simulink library "CryoDetLibCMB"  (R2016b)
settings: Solver=VariableStepAuto  StartTime=0.0  StopTime=10.0  RelTol=1e-3
undefined symbols (not defined in the file): A, B, C, D, Fadc, Fclk, PCIN, xlipgetpartsetting
libraries: xbsIndex_r4 x640, CryoDetLibCMB x81, CryoDetLib x2, simulink x1
(part 6 of 12)

== system CryoDetLibCMB/DDS 8ch ==
  note: don't worry about matching latency here, will do downstream
  note: 8 Channel DDS
      | Given its channel ID, takes instantaneous frequency for this channel of each band and generates phase and I&Q
      | interleaved over 8 bands
      | Frequency RAM is updated asynchronously to operation
  note: Phase Accumulator
      | (8 Channels)
  note: Frequency RAM
  note: Sinc/Cos Generator
  valid : Inport
  freqWord : Inport  Port=2
  index : Inport  Port=3
  ch : Inport  Port=4
  AddSub : xbsIndex_r4/AddSub  mode=Addition  use_carryin=off  use_carryout=off  en=off  latency=3  precision=User Defined  arith_type=Unsigned  n_bits=24  bin_pt=24  quantization=Truncate  overflow=Wrap  use_behavioral_HDL=off  hw_selection=Fabric  pipelined=off  dbl_ovrd=off  block_type=addsub
  BitBasher : xbsIndex_r4/BitBasher  bitexpr=|  display_expr=off  sr_1=tmux  arith_type1=Unsigned  bin_pt1=0  sr_2=subband  arith_type2=Unsigned  bin_pt2=0  sr_3=3  arith_type3=Unsigned  bin_pt3=0  sr_4=4  arith_type4=Unsigned  bin_pt4=0  dbl_ovrd=off  block_type=bitbasher
      | tmux = {in[6:4]}
      | subband = {in[3:0]}
  BitBasher1 : xbsIndex_r4/BitBasher  bitexpr=|  display_expr=off  sr_1=ch  arith_type1=Unsigned  bin_pt1=0  sr_2=amp  arith_type2=Unsigned  bin_pt2=0  sr_3=3  arith_type3=Unsigned  bin_pt3=0  sr_4=4  arith_type4=Unsigned  bin_pt4=0  dbl_ovrd=off  block_type=bitbasher
      | ch = {in[6:4]}
      | amp = {in[3:0]}
  BitBasher2 : xbsIndex_r4/BitBasher  bitexpr=|  display_expr=off  sr_1=freq  arith_type1=Unsigned  bin_pt1=24  sr_2=amp  arith_type2=Unsigned  bin_pt2=0  sr_3=3  arith_type3=Unsigned  bin_pt3=0  sr_4=4  arith_type4=Unsigned  bin_pt4=0  dbl_ovrd=off  block_type=bitbasher
      | freq = {in[23:0]}
      | amp = {in[27:24]}
  BitBasher3 : xbsIndex_r4/BitBasher  bitexpr=out = {ch, amp}  display_expr=off  sr_1=out  arith_type1=Unsigned  bin_pt1=0  sr_2=amp  arith_type2=Unsigned  bin_pt2=0  sr_3=3  arith_type3=Unsigned  bin_pt3=0  sr_4=4  arith_type4=Unsigned  bin_pt4=0  dbl_ovrd=off  block_type=bitbasher
  BitBasher4 : xbsIndex_r4/BitBasher  bitexpr=|  display_expr=off  sr_1=ch  arith_type1=Unsigned  bin_pt1=0  sr_2=amp  arith_type2=Unsigned  bin_pt2=0  sr_3=3  arith_type3=Unsigned  bin_pt3=0  sr_4=4  arith_type4=Unsigned  bin_pt4=0  dbl_ovrd=off  block_type=bitbasher
      | ch = {in[6:4]}
      | amp = {in[3:0]}
  Bus Creator : BusCreator  Inputs=3
  Convert : xbsIndex_r4/Convert  gui_display_data_type=Fixed-point  arith_type=Unsigned  n_bits=14  bin_pt=14  float_type=Single  exp_bits=8  fraction_bits=24  quantization=Truncate  overflow=Wrap  en=off  latency=1  pipeline=off  dbl_ovrd=off  block_type=convert
  Counter : xbsIndex_r4/Counter  cnt_type=Free Running  cnt_to=Inf  operation=Up  start_count=0  cnt_by_val=1  arith_type=Unsigned  n_bits=3  bin_pt=0  load_pin=off  rst=off  en=on  explicit_period=off  period=1  use_behavioral_HDL=off  implementation=Fabric  dbl_ovrd=off  block_type=counter
  "DDS Compiler 6.0 " : xbsIndex_r4/DDS Compiler 6.0   partspresent=SIN_COS_LUT_only  dds_clock_rate=100  channels=1  mode_of_operation=Standard  modulus=9  parameter_entry=System_Parameters  spurious_free_dynamic_range=45  frequency_resolution=0.4  noise_shaping=None  phase_width=14  output_width=16  output_selection=Sine_and_Cosine  negative_sine=off  negative_cosine=off  amplitude_mode=Full_Range  memory_type=Auto  optimization_goal=Auto  dsp48_use=Minimal  resync=off  latency_configuration=Auto  latency=1  has_phase_out=off  has_aclken=off  has_aresetn=off  explicit_period=off  period=1  data_has_tlast=Not_Required  has_tready=off  s_phase_has_tuser=User_Field  m_data_has_tuser=User_Field  m_phase_has_tuser=Not_Required  s_phase_tuser_width=7  output_form=Twos_Complement  s_config_sync_mode=On_Vector  phase_increment=Streaming  output_frequency1=0  output_frequency2=0  output_frequency3=0  output_frequency4=0  output_frequency5=0  output_frequency6=0  output_frequency7=0  output_frequency8=0  output_frequency9=0  output_frequency10=0  output_frequency11=0  output_frequency12=0  output_frequency13=0  output_frequency14=0  output_frequency15=0  output_frequency16=0  pinc1='0'  pinc2='0'  pinc3='0'  pinc4='0'  pinc5='0'  pinc6='0'  pinc7='0'  pinc8='0'  pinc9='0'  pinc10='0'  pinc11='0'  pinc12='0'  pinc13='0'  pinc14='0'  pinc15='0'  pinc16='0'  phase_offset=Streaming  phase_offset_angles1=0  phase_offset_angles2=0  phase_offset_angles3=0  phase_offset_angles4=0  phase_offset_angles5=0  phase_offset_angles6=0  phase_offset_angles7=0  phase_offset_angles8=0  phase_offset_angles9=0  phase_offset_angles10=0  phase_offset_angles11=0  phase_offset_angles12=0  phase_offset_angles13=0  phase_offset_angles14=0  phase_offset_angles15=0  phase_offset_angles16=0  poff1='0'  poff2='0'  poff3='0'  poff4='0'  poff5='0'  poff6='0'  poff7='0'  poff8='0'  poff9='0'  poff10='0'  poff11='0'  poff12='0'  poff13='0'  poff14='0'  poff15='0'  poff16='0'  trim_axipin_name=on  simulation_type=hybrid_sim  simulation_model=sysgen:xddsv6_0_cmodel  data_path_portlist={ 's_axis_config_tdata_poff', 's_axis_config_tdata_chan0_poff', 's_axis_config_tdata_pinc', 's_axis_config_tdata_chan0_pinc', 's_axis_phase_tdata_resync', 's_axis_phase_tdata_chan0_resync', 's_axis_phase_tdata_poff', 's_axis_phase_tdata_chan0_poff', 's_axis_phase_tdata_pinc', 's_axis_phase_tdata_chan0_pinc', 's_axis_phase_tdata_phase_in', 'm_axis_data_tdata_sine', 'm_axis_data_tdata_chan0_sine', 'm_axis_data_tdata_cosine', 'm_axis_data_tdata_chan0_cosine', 'm_axis_phase_tdata_phase_out', 'm_axis_phase_tdata_chan0_phase_out'}  por_mode=false  gui_behaviour=Sysgen  ip_name=DDS Compiler  ip_version=6.0  dsptool_ready=true  wrapper_available=true  port_translation_map={ 'aclken' => 'en', 'aresetn' => 'rst' }  ipcore_usecache=true  ipcore_useipmodelcache=true  ipcore_xco_need_fpga_part=true  ipcore_verbose=false  block_type=dds_compiler_v6_0
  Delay : xbsIndex_r4/Delay  rst=off  infoeditControl=Selection of Reset will increase slice count due to use of real FFs and instead of SRLs  en=off  latency=5  reg_retiming=off  dbl_ovrd=off  block_type=delay
  Delay1 : xbsIndex_r4/Delay  rst=off  infoeditControl=Selection of Reset will increase slice count due to use of real FFs and instead of SRLs  en=off  latency=4  reg_retiming=off  dbl_ovrd=off  block_type=delay
  Delay2 : xbsIndex_r4/Delay  rst=off  infoeditControl=Selection of Reset will increase slice count due to use of real FFs and instead of SRLs  en=off  latency=2  reg_retiming=off  dbl_ovrd=off  block_type=delay
  Delay4 : xbsIndex_r4/Delay  rst=off  infoeditControl=Selection of Reset will increase slice count due to use of real FFs and instead of SRLs  en=off  latency=6  reg_retiming=off  dbl_ovrd=off  block_type=delay
  Dual Port RAM : xbsIndex_r4/Dual Port RAM  depth=8  initVector=0  distributed_mem=Distributed memory  init_a=0  init_b=0  rst_a=off  rst_b=off  en_a=off  en_b=off  latency=1  write_mode_A=Read After Write  write_mode_B=Read After Write  optimize=Area  dbl_ovrd=off  block_type=dpram
  Register{,1..2,6} (4 alike) : xbsIndex_r4/Register  init=0  rst=off  en=off  dbl_ovrd=off  block_type=register
  Register3 : xbsIndex_r4/Register  init=0  rst=off  en=on  dbl_ovrd=off  block_type=register
  Register4 : xbsIndex_r4/Register  init=0  rst=off  en=on  dbl_ovrd=off  block_type=register
  Register5 : xbsIndex_r4/Register  init=0  rst=off  en=on  dbl_ovrd=off  block_type=register
  Relational : xbsIndex_r4/Relational  mode=a=b  op_type=Bool  en=off  latency=1  dbl_ovrd=off  block_type=relational
  Terminator : Terminator
  valid1 : InportShadow
  valid_o : Outport
  Q : Outport  Port=2
  I : Outport  Port=3
  amp_o : Outport  Port=4
  ch_o : Outport  Port=5
  phaseBus : Outport  Port=6
  wires:
  BitBasher1/1 -> Bus Creator/3  "ch"
  BitBasher4/2 -> amp_o/1
  "DDS Compiler 6.0 "/4 -> Register5/1  "INDX"
  "DDS Compiler 6.0 "/3 -> Register4/1  "I"
  Counter/1 -> Dual Port RAM/4, Delay2/1
  valid1/1 -> Delay4/1
  valid/1 -> Counter/1
  Delay4/1 -> Bus Creator/1, "DDS Compiler 6.0 "/1  "valid"
  "DDS Compiler 6.0 "/1 -> Register2/1, Register5/2, Register4/2, Register3/2  "valid"
  "DDS Compiler 6.0 "/2 -> Register3/1  "Q"
  Register1/1 -> Dual Port RAM/2
  Register/1 -> Dual Port RAM/1
  Delay1/1 -> BitBasher1/1, "DDS Compiler 6.0 "/3  "ch"
  Dual Port RAM/1 -> Terminator/1
  Convert/1 -> Bus Creator/2, "DDS Compiler 6.0 "/2  "phase"
  AddSub/1 -> Convert/1, Delay/1
  ch/1 -> BitBasher/1
  Delay/1 -> AddSub/1
  Relational/1 -> Dual Port RAM/3
  BitBasher/1 -> Register/1
  BitBasher/2 -> Relational/1
  index/1 -> Relational/2
  Register4/1 -> I/1  "I"
  Register3/1 -> Q/1  "Q"
  Register2/1 -> valid_o/1  "valid"
  freqWord/1 -> Register1/1
  Dual Port RAM/2 -> Register6/1
  BitBasher2/1 -> AddSub/2
  BitBasher2/2 -> BitBasher3/1
  BitBasher3/1 -> Delay1/1
  Register5/1 -> BitBasher4/1  "INDX"
  BitBasher4/1 -> ch_o/1
  Register6/1 -> BitBasher2/1
  Delay2/1 -> BitBasher3/2
  Bus Creator/1 -> phaseBus/1

== system CryoDetLibCMB/DDS 8ch taylor series corrected ==
  note: Taylor series corrected - use 0.5 BRAM (18 bit storage, 2^10 points), 3DSP
  note: Frequency RAM
  note: Phase Accumulator
      | (8 Channels)
  note: 8 Channel DDS
      | Given its channel ID, takes instantaneous frequency for this channel of each band and generates phase and I&Q
      | interleaved over 8 bands
      | Frequency RAM is updated asynchronously to operation
  note: don't worry about matching latency here, will do downstream
  valid : Inport
  rst : Inport  Port=2
  freqWord : Inport  Port=3
  index : Inport  Port=4
  ch : Inport  Port=5
  BitBasher : xbsIndex_r4/BitBasher  bitexpr=|  display_expr=off  sr_1=tmux  arith_type1=Unsigned  bin_pt1=0  sr_2=subband  arith_type2=Unsigned  bin_pt2=0  sr_3=3  arith_type3=Unsigned  bin_pt3=0  sr_4=4  arith_type4=Unsigned  bin_pt4=0  dbl_ovrd=off  block_type=bitbasher
      | tmux = {in[6:4]}
      | subband = {in[3:0]}
  BitBasher1 : xbsIndex_r4/BitBasher  bitexpr=|  display_expr=off  sr_1=ch  arith_type1=Unsigned  bin_pt1=0  sr_2=amp  arith_type2=Unsigned  bin_pt2=0  sr_3=3  arith_type3=Unsigned  bin_pt3=0  sr_4=4  arith_type4=Unsigned  bin_pt4=0  dbl_ovrd=off  block_type=bitbasher
      | ch = {in[6:4]}
      | amp = {in[3:0]}
  BitBasher2 : xbsIndex_r4/BitBasher  bitexpr=|  display_expr=off  sr_1=freq  arith_type1=Unsigned  bin_pt1=24  sr_2=amp  arith_type2=Unsigned  bin_pt2=0  sr_3=3  arith_type3=Unsigned  bin_pt3=0  sr_4=4  arith_type4=Unsigned  bin_pt4=0  dbl_ovrd=off  block_type=bitbasher
      | freq = {in[23:0]}
      | amp = {in[27:24]}
  BitBasher3 : xbsIndex_r4/BitBasher  bitexpr=out = {ch, amp}  display_expr=off  sr_1=out  arith_type1=Unsigned  bin_pt1=0  sr_2=amp  arith_type2=Unsigned  bin_pt2=0  sr_3=3  arith_type3=Unsigned  bin_pt3=0  sr_4=4  arith_type4=Unsigned  bin_pt4=0  dbl_ovrd=off  block_type=bitbasher
  BitBasher4 : xbsIndex_r4/BitBasher  bitexpr=|  display_expr=off  sr_1=ch  arith_type1=Unsigned  bin_pt1=0  sr_2=amp  arith_type2=Unsigned  bin_pt2=0  sr_3=3  arith_type3=Unsigned  bin_pt3=0  sr_4=4  arith_type4=Unsigned  bin_pt4=0  dbl_ovrd=off  block_type=bitbasher
      | ch = {in[6:4]}
      | amp = {in[3:0]}
  BitBasher5 : xbsIndex_r4/BitBasher  bitexpr=phase = {in[23:8]}  display_expr=off  sr_1=phase  arith_type1="Signed  (2's comp)"  bin_pt1=15  sr_2=amp  arith_type2=Unsigned  bin_pt2=0  sr_3=3  arith_type3=Unsigned  bin_pt3=0  sr_4=4  arith_type4=Unsigned  bin_pt4=0  dbl_ovrd=off  block_type=bitbasher
  Bus Creator : BusCreator  Inputs=3
  Counter : xbsIndex_r4/Counter  cnt_type=Free Running  cnt_to=Inf  operation=Up  start_count=0  cnt_by_val=1  arith_type=Unsigned  n_bits=3  bin_pt=0  load_pin=off  rst=on  en=on  explicit_period=off  period=1  use_behavioral_HDL=off  implementation=Fabric  dbl_ovrd=off  block_type=counter
  DDS Compiler 6.0 1 : xbsIndex_r4/DDS Compiler 6.0   partspresent=Phase_Generator_only  dds_clock_rate=100  channels=8  mode_of_operation=Standard  modulus=9  parameter_entry=System_Parameters  spurious_free_dynamic_range=45  frequency_resolution=0.4  noise_shaping=None  phase_width=24  output_width=3  output_selection=Sine_and_Cosine  negative_sine=off  negative_cosine=off  amplitude_mode=Full_Range  memory_type=Auto  optimization_goal=Auto  dsp48_use=Minimal  resync=off  latency_configuration=Auto  latency=1  has_phase_out=on  has_aclken=off  has_aresetn=on  explicit_period=off  period=1  data_has_tlast=Not_Required  has_tready=off  s_phase_has_tuser=User_Field  m_data_has_tuser=Not_Required  m_phase_has_tuser=User_Field  s_phase_tuser_width=7  output_form=Twos_Complement  s_config_sync_mode=On_Vector  phase_increment=Streaming  output_frequency1=0  output_frequency2=0  output_frequency3=0  output_frequency4=0  output_frequency5=0  output_frequency6=0  output_frequency7=0  output_frequency8=0  output_frequency9=0  output_frequency10=0  output_frequency11=0  output_frequency12=0  output_frequency13=0  output_frequency14=0  output_frequency15=0  output_frequency16=0  pinc1='0'  pinc2='0'  pinc3='0'  pinc4='0'  pinc5='0'  pinc6='0'  pinc7='0'  pinc8='0'  pinc9='0'  pinc10='0'  pinc11='0'  pinc12='0'  pinc13='0'  pinc14='0'  pinc15='0'  pinc16='0'  phase_offset=None  phase_offset_angles1=0  phase_offset_angles2=0  phase_offset_angles3=0  phase_offset_angles4=0  phase_offset_angles5=0  phase_offset_angles6=0  phase_offset_angles7=0  phase_offset_angles8=0  phase_offset_angles9=0  phase_offset_angles10=0  phase_offset_angles11=0  phase_offset_angles12=0  phase_offset_angles13=0  phase_offset_angles14=0  phase_offset_angles15=0  phase_offset_angles16=0  poff1='0'  poff2='0'  poff3='0'  poff4='0'  poff5='0'  poff6='0'  poff7='0'  poff8='0'  poff9='0'  poff10='0'  poff11='0'  poff12='0'  poff13='0'  poff14='0'  poff15='0'  poff16='0'  trim_axipin_name=on  simulation_type=hybrid_sim  simulation_model=sysgen:xddsv6_0_cmodel  data_path_portlist={ 's_axis_config_tdata_poff', 's_axis_config_tdata_chan0_poff', 's_axis_config_tdata_pinc', 's_axis_config_tdata_chan0_pinc', 's_axis_phase_tdata_resync', 's_axis_phase_tdata_chan0_resync', 's_axis_phase_tdata_poff', 's_axis_phase_tdata_chan0_poff', 's_axis_phase_tdata_pinc', 's_axis_phase_tdata_chan0_pinc', 's_axis_phase_tdata_phase_in', 'm_axis_data_tdata_sine', 'm_axis_data_tdata_chan0_sine', 'm_axis_data_tdata_cosine', 'm_axis_data_tdata_chan0_cosine', 'm_axis_phase_tdata_phase_out', 'm_axis_phase_tdata_chan0_phase_out'}  por_mode=false  gui_behaviour=Sysgen  ip_name=DDS Compiler  ip_version=6.0  dsptool_ready=true  wrapper_available=true  port_translation_map={ 'aclken' => 'en', 'aresetn' => 'rst' }  ipcore_usecache=true  ipcore_useipmodelcache=true  ipcore_xco_need_fpga_part=true  ipcore_verbose=false  block_type=dds_compiler_v6_0
  DDS Compiler 6.0 2 : xbsIndex_r4/DDS Compiler 6.0   partspresent=SIN_COS_LUT_only  dds_clock_rate=100  channels=1  mode_of_operation=Standard  modulus=9  parameter_entry=System_Parameters  spurious_free_dynamic_range=45  frequency_resolution=0.4  noise_shaping=Taylor_Series_Corrected  phase_width=24  output_width=18  output_selection=Sine_and_Cosine  negative_sine=off  negative_cosine=off  amplitude_mode=Full_Range  memory_type=Auto  optimization_goal=Area  dsp48_use=Minimal  resync=off  latency_configuration=Auto  latency=1  has_phase_out=off  has_aclken=off  has_aresetn=off  explicit_period=off  period=1  data_has_tlast=Not_Required  has_tready=off  s_phase_has_tuser=User_Field  m_data_has_tuser=User_Field  m_phase_has_tuser=Not_Required  s_phase_tuser_width=7  output_form=Twos_Complement  s_config_sync_mode=On_Vector  phase_increment=Streaming  output_frequency1=0  output_frequency2=0  output_frequency3=0  output_frequency4=0  output_frequency5=0  output_frequency6=0  output_frequency7=0  output_frequency8=0  output_frequency9=0  output_frequency10=0  output_frequency11=0  output_frequency12=0  output_frequency13=0  output_frequency14=0  output_frequency15=0  output_frequency16=0  pinc1='0'  pinc2='0'  pinc3='0'  pinc4='0'  pinc5='0'  pinc6='0'  pinc7='0'  pinc8='0'  pinc9='0'  pinc10='0'  pinc11='0'  pinc12='0'  pinc13='0'  pinc14='0'  pinc15='0'  pinc16='0'  phase_offset=Streaming  phase_offset_angles1=0  phase_offset_angles2=0  phase_offset_angles3=0  phase_offset_angles4=0  phase_offset_angles5=0  phase_offset_angles6=0  phase_offset_angles7=0  phase_offset_angles8=0  phase_offset_angles9=0  phase_offset_angles10=0  phase_offset_angles11=0  phase_offset_angles12=0  phase_offset_angles13=0  phase_offset_angles14=0  phase_offset_angles15=0  phase_offset_angles16=0  poff1='0'  poff2='0'  poff3='0'  poff4='0'  poff5='0'  poff6='0'  poff7='0'  poff8='0'  poff9='0'  poff10='0'  poff11='0'  poff12='0'  poff13='0'  poff14='0'  poff15='0'  poff16='0'  trim_axipin_name=on  simulation_type=hybrid_sim  simulation_model=sysgen:xddsv6_0_cmodel  data_path_portlist={ 's_axis_config_tdata_poff', 's_axis_config_tdata_chan0_poff', 's_axis_config_tdata_pinc', 's_axis_config_tdata_chan0_pinc', 's_axis_phase_tdata_resync', 's_axis_phase_tdata_chan0_resync', 's_axis_phase_tdata_poff', 's_axis_phase_tdata_chan0_poff', 's_axis_phase_tdata_pinc', 's_axis_phase_tdata_chan0_pinc', 's_axis_phase_tdata_phase_in', 'm_axis_data_tdata_sine', 'm_axis_data_tdata_chan0_sine', 'm_axis_data_tdata_cosine', 'm_axis_data_tdata_chan0_cosine', 'm_axis_phase_tdata_phase_out', 'm_axis_phase_tdata_chan0_phase_out'}  por_mode=false  gui_behaviour=Sysgen  ip_name=DDS Compiler  ip_version=6.0  dsptool_ready=true  wrapper_available=true  port_translation_map={ 'aclken' => 'en', 'aresetn' => 'rst' }  ipcore_usecache=true  ipcore_useipmodelcache=true  ipcore_xco_need_fpga_part=true  ipcore_verbose=false  block_type=dds_compiler_v6_0
  Delay2 : xbsIndex_r4/Delay  rst=off  infoeditControl=Selection of Reset will increase slice count due to use of real FFs and instead of SRLs  en=off  latency=2  reg_retiming=off  dbl_ovrd=off  block_type=delay
  Delay4 : xbsIndex_r4/Delay  rst=off  infoeditControl=Selection of Reset will increase slice count due to use of real FFs and instead of SRLs  en=off  latency=2  reg_retiming=off  dbl_ovrd=off  block_type=delay
  Dual Port RAM : xbsIndex_r4/Dual Port RAM  depth=8  initVector=0  distributed_mem=Distributed memory  init_a=0  init_b=0  rst_a=off  rst_b=off  en_a=off  en_b=off  latency=1  write_mode_A=Read After Write  write_mode_B=Read After Write  optimize=Area  dbl_ovrd=off  block_type=dpram
  Inverter : xbsIndex_r4/Inverter  en=off  latency=1  dbl_ovrd=off  block_type=inv
  Register{,1..2,6} (4 alike) : xbsIndex_r4/Register  init=0  rst=off  en=off  dbl_ovrd=off  block_type=register
  Register3 : xbsIndex_r4/Register  init=0  rst=off  en=on  dbl_ovrd=off  block_type=register
  Register4 : xbsIndex_r4/Register  init=0  rst=off  en=on  dbl_ovrd=off  block_type=register
  Register5 : xbsIndex_r4/Register  init=0  rst=off  en=on  dbl_ovrd=off  block_type=register
  Relational : xbsIndex_r4/Relational  mode=a=b  op_type=Bool  en=off  latency=1  dbl_ovrd=off  block_type=relational
  Terminator : Terminator
  Terminator1 : Terminator
  Terminator2 : Terminator
  tuser : xbsIndex_r4/Constant  const=0  gui_display_data_type=Boolean  arith_type=Boolean  n_bits=1  bin_pt=0  preci_type=Single  exp_width=8  frac_width=24  explicit_period=off  period=1  equ=P=C  opselect=C  inp2=PCIN>>17  opr=+  inp1=P  carry=CIN  dbl_ovrd=off  block_type=constant
  valid1 : InportShadow
  valid_o : Outport
  Q : Outport  Port=2
  I : Outport  Port=3
  amp_o : Outport  Port=4
  ch_o : Outport  Port=5
  phaseBus : Outport  Port=6
  wires:
  Inverter/1 -> DDS Compiler 6.0 1/5
  valid/1 -> Counter/2
  rst/1 -> Counter/1, Inverter/1
  BitBasher5/1 -> Bus Creator/2  "phase"
  Bus Creator/1 -> phaseBus/1
  Delay2/1 -> BitBasher3/2
  Register6/1 -> BitBasher2/1
  BitBasher4/1 -> ch_o/1
  Register5/1 -> BitBasher4/1  "INDX"
  BitBasher2/2 -> BitBasher3/1
  Dual Port RAM/2 -> Register6/1
  freqWord/1 -> Register1/1
  Register2/1 -> valid_o/1  "valid"
  Register3/1 -> Q/1  "Q"
  Register4/1 -> I/1  "I"
  index/1 -> Relational/2
  BitBasher/2 -> Relational/1
  BitBasher/1 -> Register/1
  Relational/1 -> Dual Port RAM/3
  ch/1 -> BitBasher/1
  Dual Port RAM/1 -> Terminator/1
  Register/1 -> Dual Port RAM/1
  Register1/1 -> Dual Port RAM/2
  DDS Compiler 6.0 2/2 -> Register3/1  "Q"
  DDS Compiler 6.0 2/1 -> Register5/2, Register4/2, Register3/2, Register2/1  "valid"
  valid1/1 -> Delay4/1
  Counter/1 -> Delay2/1, Dual Port RAM/4
  DDS Compiler 6.0 2/3 -> Register4/1  "I"
  DDS Compiler 6.0 2/4 -> Register5/1  "INDX"
  BitBasher4/2 -> amp_o/1
  BitBasher1/1 -> Bus Creator/3  "ch"
  DDS Compiler 6.0 1/1 -> Bus Creator/1, DDS Compiler 6.0 2/1  "valid"
  BitBasher2/1 -> DDS Compiler 6.0 1/2
  BitBasher3/1 -> DDS Compiler 6.0 1/4
  Delay4/1 -> DDS Compiler 6.0 1/1  "valid"
  DDS Compiler 6.0 1/2 -> DDS Compiler 6.0 2/2, BitBasher5/1  "phase"
  DDS Compiler 6.0 1/3 -> DDS Compiler 6.0 2/3, BitBasher1/1  "tyser"
  tuser/1 -> DDS Compiler 6.0 1/3
  DDS Compiler 6.0 1/4 -> Terminator1/1
  DDS Compiler 6.0 1/5 -> Terminator2/1

== system CryoDetLibCMB/DDS Mixer ==
  In : Inport
  freqBus : Inport  Port=2
  index : Inport  Port=3
  Bus Creator1 : BusCreator  Inputs=4
  Bus Creator2 : BusCreator  Inputs=5
  Bus Selector1 : BusSelector  OutputSignals=valid,Q,I,amp,ch
  Bus Selector2 : BusSelector  OutputSignals=valid
  Bus Selector : BusSelector  OutputSignals=freqWord,ch
  DDS 8ch : CryoDetLibCMB/DDS 8ch
  IQ_scale : CryoDetLibCMB/IQ_scale
  mixer : Subsystem
  tones : Outport
  downconvert : Outport  Port=2
  phase : Outport  Port=3
  wires:
  Bus Selector/1 -> DDS 8ch/2  "<freqWord>"
  Bus Selector1/5 -> IQ_scale/5  "<ch>"
  Bus Selector1/4 -> IQ_scale/4  "<amp>"
  DDS 8ch/4 -> Bus Creator2/4  "amp"
  DDS 8ch/5 -> Bus Creator2/5  "ch"
  In/1 -> mixer/2(In2), Bus Selector2/1
  freqBus/1 -> Bus Selector/1
  Bus Selector2/1 -> DDS 8ch/1  "<valid>"
  index/1 -> DDS 8ch/3
  IQ_scale/1 -> Bus Creator1/1  "valid"
  IQ_scale/2 -> Bus Creator1/2  "Q"
  IQ_scale/3 -> Bus Creator1/3  "I"
  IQ_scale/4 -> Bus Creator1/4  "ch"
  Bus Creator1/1 -> tones/1
  DDS 8ch/3 -> Bus Creator2/3  "I"
  DDS 8ch/1 -> Bus Creator2/1  "valid"
  DDS 8ch/2 -> Bus Creator2/2  "Q"
  Bus Creator2/1 -> mixer/1(In1), Bus Selector1/1
  Bus Selector1/3 -> IQ_scale/3  "<I>"
  Bus Selector1/2 -> IQ_scale/2  "<Q>"
  Bus Selector1/1 -> IQ_scale/1  "<valid>"
  Bus Selector/2 -> DDS 8ch/4  "<ch>"
  mixer/1(downmix) -> downconvert/1  "valid"
  mixer/2(phaseBus_o) -> phase/1
  DDS 8ch/6 -> mixer/3(phaseBus)

== system CryoDetLibCMB/DDS Mixer taylor series corrected ==
  rst : Inport
  In : Inport  Port=2
  freqBus : Inport  Port=3
  index : Inport  Port=4
  Bus Creator1 : BusCreator  Inputs=4
  Bus Creator2 : BusCreator  Inputs=5
  Bus Selector1 : BusSelector  OutputSignals=valid,Q,I,amp,ch
  Bus Selector2 : BusSelector  OutputSignals=valid
  Bus Selector : BusSelector  OutputSignals=freqWord,ch
  DDS 8ch taylor series corrected : CryoDetLibCMB/DDS 8ch taylor series corrected
  IQ_scale : CryoDetLibCMB/IQ_scale
  mixer : Subsystem
  tones : Outport
  downconvert : Outport  Port=2
  phase : Outport  Port=3
  wires:
  rst/1 -> DDS 8ch taylor series corrected/2
  Bus Selector/1 -> DDS 8ch taylor series corrected/3  "<freqWord>"
  Bus Selector1/5 -> IQ_scale/5  "<ch>"
  Bus Selector1/4 -> IQ_scale/4  "<amp>"
  DDS 8ch taylor series corrected/4 -> Bus Creator2/4  "amp"
  DDS 8ch taylor series corrected/5 -> Bus Creator2/5  "ch"
  In/1 -> mixer/2(In2), Bus Selector2/1
  freqBus/1 -> Bus Selector/1
  Bus Selector2/1 -> DDS 8ch taylor series corrected/1  "<valid>"
  index/1 -> DDS 8ch taylor series corrected/4
  IQ_scale/1 -> Bus Creator1/1  "valid"
  IQ_scale/2 -> Bus Creator1/2  "Q"
  IQ_scale/3 -> Bus Creator1/3  "I"
  IQ_scale/4 -> Bus Creator1/4  "ch"
  Bus Creator1/1 -> tones/1
  DDS 8ch taylor series corrected/3 -> Bus Creator2/3  "I"
  DDS 8ch taylor series corrected/1 -> Bus Creator2/1  "valid"
  DDS 8ch taylor series corrected/2 -> Bus Creator2/2  "Q"
  Bus Creator2/1 -> mixer/1(In1), Bus Selector1/1
  Bus Selector1/3 -> IQ_scale/3  "<I>"
  Bus Selector1/2 -> IQ_scale/2  "<Q>"
  Bus Selector1/1 -> IQ_scale/1  "<valid>"
  Bus Selector/2 -> DDS 8ch taylor series corrected/5  "<ch>"
  mixer/1(downmix) -> downconvert/1  "valid"
  mixer/2(phaseBus_o) -> phase/1
  DDS 8ch taylor series corrected/6 -> mixer/3(phaseBus)

== system CryoDetLibCMB/DDS Mixer_empty ==
  In : Inport
  freqBus : Inport  Port=2
  index : Inport  Port=3
  Bus Creator : BusCreator  Inputs=3
  Bus Creator1 : BusCreator  Inputs=4
  Bus Creator2 : BusCreator  Inputs=4
  Constant : xbsIndex_r4/Constant  const=0  gui_display_data_type=Fixed-point  arith_type=Signed (2's comp)  n_bits=18  bin_pt=17  preci_type=Single  exp_width=8  frac_width=24  explicit_period=on  period=2/Fadc  equ=P=C  opselect=C  inp2=PCIN>>17  opr=+  inp1=P  carry=CIN  dbl_ovrd=off  block_type=constant
  Constant1 : xbsIndex_r4/Constant  const=0  gui_display_data_type=Fixed-point  arith_type=Signed (2's comp)  n_bits=18  bin_pt=17  preci_type=Single  exp_width=8  frac_width=24  explicit_period=on  period=2/Fadc  equ=P=C  opselect=C  inp2=PCIN>>17  opr=+  inp1=P  carry=CIN  dbl_ovrd=off  block_type=constant
  Constant10 : xbsIndex_r4/Constant  const=0  gui_display_data_type=Fixed-point  arith_type=Unsigned  n_bits=3  bin_pt=0  preci_type=Single  exp_width=8  frac_width=24  explicit_period=on  period=2/Fadc  equ=P=C  opselect=C  inp2=PCIN>>17  opr=+  inp1=P  carry=CIN  dbl_ovrd=off  block_type=constant
  Constant2 : xbsIndex_r4/Constant  const=0  gui_display_data_type=Boolean  arith_type=Boolean  n_bits=18  bin_pt=17  preci_type=Single  exp_width=8  frac_width=24  explicit_period=on  period=2/Fadc  equ=P=C  opselect=C  inp2=PCIN>>17  opr=+  inp1=P  carry=CIN  dbl_ovrd=off  block_type=constant
  Constant3 : xbsIndex_r4/Constant  const=0  gui_display_data_type=Fixed-point  arith_type=Unsigned  n_bits=3  bin_pt=0  preci_type=Single  exp_width=8  frac_width=24  explicit_period=on  period=2/Fadc  equ=P=C  opselect=C  inp2=PCIN>>17  opr=+  inp1=P  carry=CIN  dbl_ovrd=off  block_type=constant
  Constant4 : xbsIndex_r4/Constant  const=0  gui_display_data_type=Boolean  arith_type=Boolean  n_bits=18  bin_pt=17  preci_type=Single  exp_width=8  frac_width=24  explicit_period=on  period=2/Fadc  equ=P=C  opselect=C  inp2=PCIN>>17  opr=+  inp1=P  carry=CIN  dbl_ovrd=off  block_type=constant
  Constant5 : xbsIndex_r4/Constant  const=0  gui_display_data_type=Fixed-point  arith_type=Unsigned  n_bits=3  bin_pt=0  preci_type=Single  exp_width=8  frac_width=24  explicit_period=on  period=2/Fadc  equ=P=C  opselect=C  inp2=PCIN>>17  opr=+  inp1=P  carry=CIN  dbl_ovrd=off  block_type=constant
  Constant6 : xbsIndex_r4/Constant  const=0  gui_display_data_type=Fixed-point  arith_type=Unsigned  n_bits=14  bin_pt=14  preci_type=Single  exp_width=8  frac_width=24  explicit_period=on  period=2/Fadc  equ=P=C  opselect=C  inp2=PCIN>>17  opr=+  inp1=P  carry=CIN  dbl_ovrd=off  block_type=constant
  Constant7 : xbsIndex_r4/Constant  const=0  gui_display_data_type=Fixed-point  arith_type=Signed (2's comp)  n_bits=18  bin_pt=16  preci_type=Single  exp_width=8  frac_width=24  explicit_period=on  period=2/Fadc  equ=P=C  opselect=C  inp2=PCIN>>17  opr=+  inp1=P  carry=CIN  dbl_ovrd=off  block_type=constant
  Constant8 : xbsIndex_r4/Constant  const=0  gui_display_data_type=Fixed-point  arith_type=Signed (2's comp)  n_bits=18  bin_pt=16  preci_type=Single  exp_width=8  frac_width=24  explicit_period=on  period=2/Fadc  equ=P=C  opselect=C  inp2=PCIN>>17  opr=+  inp1=P  carry=CIN  dbl_ovrd=off  block_type=constant
  Constant9 : xbsIndex_r4/Constant  const=0  gui_display_data_type=Boolean  arith_type=Boolean  n_bits=18  bin_pt=17  preci_type=Single  exp_width=8  frac_width=24  explicit_period=on  period=2/Fadc  equ=P=C  opselect=C  inp2=PCIN>>17  opr=+  inp1=P  carry=CIN  dbl_ovrd=off  block_type=constant
  tones : Outport
  downconvert : Outport  Port=2
  phase : Outport  Port=3
  wires:
  Bus Creator2/1 -> downconvert/1  "valid"
  Bus Creator1/1 -> tones/1
  Constant3/1 -> Bus Creator1/4  "ch"
  Constant1/1 -> Bus Creator1/3  "I"
  Constant/1 -> Bus Creator1/2  "Q"
  Constant2/1 -> Bus Creator1/1  "valid"
  Bus Creator/1 -> phase/1
  Constant4/1 -> Bus Creator/1  "valid"
  Constant5/1 -> Bus Creator/2  "ch"
  Constant6/1 -> Bus Creator/3  "phase"
  Constant10/1 -> Bus Creator2/4  "ch"
  Constant8/1 -> Bus Creator2/3  "I"
  Constant7/1 -> Bus Creator2/2  "Q"
  Constant9/1 -> Bus Creator2/1  "valid"

== system CryoDetLibCMB/Demod Debug Scope ==
  note: Debug Demodulation
  demod : Inport
  freq : Inport  Port=2
  Complex to Magnitude-Angle : ComplexToMagnitudeAngle  Output=Magnitude
  Demux1 : Demux
  Gain : Gain  Gain=Fclk
  Gateway Out{1,3..6} (5 alike) : xbsIndex_r4/Gateway Out  inherit_from_input=off  hdl_port=off  rows=1  columns=1  UseAsDAC=off  DACChannel='1'  interface=None  automatic_assignment=on  address_offset=hex2dec('00')  intf_name=''  intf_description=''  timing_constraint=None  locs_specified=off  LOCs={}  io_standard={}  block_type=gatewayout
  Mux4 : Mux  Inputs=3
  Mux5 : Mux  Inputs=2
  Real-Imag to Complex : RealImagToComplex
  block downconverter Scope : Scope  NumInputPorts=3
  wires:
  demod/1 -> Demux1/1
  Demux1/1 -> Gateway Out3/1
  Demux1/2 -> Gateway Out4/1
  Demux1/3 -> Gateway Out5/1
  Demux1/4 -> Gateway Out6/1
  Gateway Out6/1 -> Mux5/2
  Gateway Out5/1 -> Mux5/1
  Gateway Out4/1 -> Mux4/2, Real-Imag to Complex/1
  Gateway Out3/1 -> Mux4/1, Real-Imag to Complex/2
  Mux4/1 -> block downconverter Scope/1
  Mux5/1 -> block downconverter Scope/2
  Complex to Magnitude-Angle/1 -> Mux4/3
  Real-Imag to Complex/1 -> Complex to Magnitude-Angle/1
  freq/1 -> Gateway Out1/1
  Gateway Out1/1 -> Gain/1
  Gain/1 -> block downconverter Scope/3

== system CryoDetLibCMB/DownSample ==
  note: DownSample with rate change given by Naxi
  In : Inport
  Down Sample : xbsIndex_r4/Down Sample  sample_ratio=Naxi  sample_phase="Last Value of Frame  (most efficient)"  en=off  rst=off  latency=1  dbl_ovrd=off  block_type=dsamp
  Register : xbsIndex_r4/Register  init=0  rst=off  en=off  dbl_ovrd=off  block_type=register
  Register1 : xbsIndex_r4/Register  init=0  rst=off  en=off  dbl_ovrd=off  block_type=register
  Out : Outport
  wires:
  Register/1 -> Register1/1
  In/1 -> Down Sample/1
  Down Sample/1 -> Register/1
  Register1/1 -> Out/1

== system CryoDetLibCMB/IQ_scale ==
  valid : Inport
  in0 : Inport  Port=2
  in1 : Inport  Port=3
  ampl : Inport  Port=4
  ch : Inport  Port=5
  amplitude_scale : CryoDetLibCMB/amplitude_scale
  amplitude_scale1 : CryoDetLibCMB/amplitude_scale
  valid_o : Outport
  out0 : Outport  Port=2
  out1 : Outport  Port=3
  ch_o : Outport  Port=4
  wires:
  amplitude_scale1/2 -> out1/1
  amplitude_scale/2 -> out0/1
  valid/1 -> amplitude_scale1/1, amplitude_scale/1
  ampl/1 -> amplitude_scale1/2, amplitude_scale/2
  in0/1 -> amplitude_scale/3
  ch/1 -> amplitude_scale1/4, amplitude_scale/4
  in1/1 -> amplitude_scale1/3
  amplitude_scale/1 -> valid_o/1
  amplitude_scale/3 -> ch_o/1

== system CryoDetLibCMB/Impulse Generator ==
  note: Parameters are:
      | width:	 pulse width (seconds)
      | Impulse:	Area of pulse = Amplitude*width
      | Period:	Pulse repetition time (seconds)
      | delay:	start time of pulse (seconds)
  Pulse Generator1 : DiscretePulseGenerator  PulseType=Time based  Amplitude=Impulse/width  Period=Period  PulseWidth=100 * width/Period  PhaseDelay=delay
  Out1 : Outport
  wires:
  Pulse Generator1/1 -> Out1/1

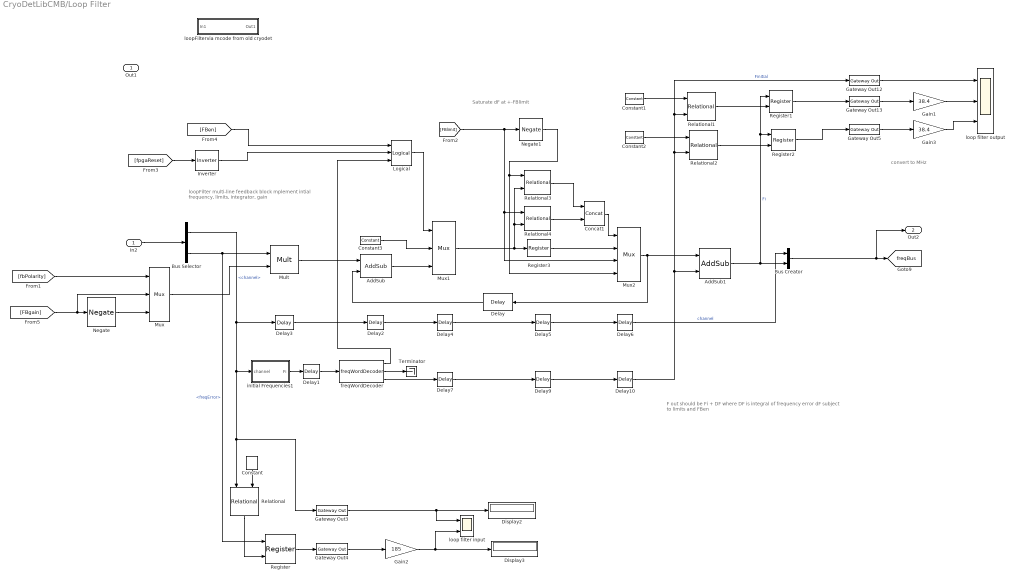
== system CryoDetLibCMB/Loop Filter ==
  note: Saturate dF at +-FBlimit
  note: convert to MHz
  note: F out should be Fi + DF
      | where DF is integral of frequency error dF subject to limits and FBen
  note: loopFilter
      | multi-line feedback block
      | mplement intial frequency, limits, integrator, gain
  In2 : Inport
  AddSub : xbsIndex_r4/AddSub  mode=Addition  use_carryin=off  use_carryout=off  en=off  latency=1  precision=User Defined  arith_type="Signed  (2's comp)"  n_bits=32  bin_pt=30  quantization=Truncate  overflow=Saturate  use_behavioral_HDL=off  hw_selection=Fabric  pipelined=off  dbl_ovrd=off  block_type=addsub
  AddSub1 : xbsIndex_r4/AddSub  mode=Addition  use_carryin=off  use_carryout=off  en=off  latency=1  precision=Full  arith_type=Unsigned  n_bits=16  bin_pt=14  quantization=Truncate  overflow=Wrap  use_behavioral_HDL=off  hw_selection=Fabric  pipelined=off  dbl_ovrd=off  block_type=addsub
  Bus Selector : BusSelector  OutputSignals=channel,freqError
  Bus Creator : BusCreator  Inputs=2
  Concat1 : xbsIndex_r4/Concat  num_inputs=2  dbl_ovrd=off  block_type=concat
  Constant : xbsIndex_r4/Constant  const=0  gui_display_data_type=Fixed-point  arith_type=Unsigned  n_bits=4  bin_pt=0  preci_type=Single  exp_width=8  frac_width=24  explicit_period=off  period=1  equ=P=C  opselect=C  inp2=PCIN>>17  opr=+  inp1=P  carry=CIN  dbl_ovrd=off  block_type=constant
  Constant1 : xbsIndex_r4/Constant  const=0  gui_display_data_type=Fixed-point  arith_type=Unsigned  n_bits=4  bin_pt=0  preci_type=Single  exp_width=8  frac_width=24  explicit_period=off  period=1  equ=P=C  opselect=C  inp2=PCIN>>17  opr=+  inp1=P  carry=CIN  dbl_ovrd=off  block_type=constant
  Constant2 : xbsIndex_r4/Constant  const=6  gui_display_data_type=Fixed-point  arith_type=Unsigned  n_bits=4  bin_pt=0  preci_type=Single  exp_width=8  frac_width=24  explicit_period=off  period=1  equ=P=C  opselect=C  inp2=PCIN>>17  opr=+  inp1=P  carry=CIN  dbl_ovrd=off  block_type=constant
  Constant3 : xbsIndex_r4/Constant  const=0  gui_display_data_type=Fixed-point  arith_type=Signed (2's comp)  n_bits=32  bin_pt=30  preci_type=Single  exp_width=8  frac_width=24  explicit_period=off  period=1  equ=P=C  opselect=C  inp2=PCIN>>17  opr=+  inp1=P  carry=CIN  dbl_ovrd=off  block_type=constant
  Delay : xbsIndex_r4/Delay  rst=off  infoeditControl=Selection of Reset will increase slice count due to use of real FFs and instead of SRLs  en=off  latency=124  reg_retiming=off  dbl_ovrd=off  block_type=delay
  Delay1 : xbsIndex_r4/Delay  rst=off  infoeditControl=Selection of Reset will increase slice count due to use of real FFs and instead of SRLs  en=off  latency=2  reg_retiming=off  dbl_ovrd=off  block_type=delay
  Delay{2,4..6,9..10} (6 alike) : xbsIndex_r4/Delay  rst=off  infoeditControl=Selection of Reset will increase slice count due to use of real FFs and instead of SRLs  en=off  latency=1  reg_retiming=off  dbl_ovrd=off  block_type=delay
  Delay3 : xbsIndex_r4/Delay  rst=off  infoeditControl=Selection of Reset will increase slice count due to use of real FFs and instead of SRLs  en=off  latency=3  reg_retiming=off  dbl_ovrd=off  block_type=delay
  Delay7 : xbsIndex_r4/Delay  rst=off  infoeditControl=Selection of Reset will increase slice count due to use of real FFs and instead of SRLs  en=off  latency=2  reg_retiming=off  dbl_ovrd=off  block_type=delay
  Display2 : Display
  Display3 : Display
  Gain1 : Gain  Gain=38.4
  Gain2 : Gain  Gain=185
  Gain3 : Gain  Gain=38.4
  Gateway Out12 : xbsIndex_r4/Gateway Out  inherit_from_input=off  hdl_port=off  rows=1  columns=1  UseAsDAC=off  DACChannel='1'  interface=None  automatic_assignment=on  address_offset=hex2dec('00')  intf_name=''  intf_description=''  timing_constraint=None  locs_specified=off  LOCs={}  io_standard={}  block_type=gatewayout
  Gateway Out13 : xbsIndex_r4/Gateway Out  inherit_from_input=on  hdl_port=off  rows=1  columns=1  UseAsDAC=off  DACChannel='1'  interface=None  automatic_assignment=on  address_offset=hex2dec('00')  intf_name=''  intf_description=''  timing_constraint=None  locs_specified=off  LOCs={}  io_standard={}  block_type=gatewayout
  Gateway Out3 : xbsIndex_r4/Gateway Out  inherit_from_input=off  hdl_port=off  rows=1  columns=1  UseAsDAC=off  DACChannel='1'  interface=None  automatic_assignment=on  address_offset=hex2dec('00')  intf_name=''  intf_description=''  timing_constraint=None  locs_specified=off  LOCs={}  io_standard={}  block_type=gatewayout
  Gateway Out4 : xbsIndex_r4/Gateway Out  inherit_from_input=off  hdl_port=off  rows=1  columns=1  UseAsDAC=off  DACChannel='1'  interface=None  automatic_assignment=on  address_offset=hex2dec('00')  intf_name=''  intf_description=''  timing_constraint=None  locs_specified=off  LOCs={}  io_standard={}  block_type=gatewayout
  Gateway Out5 : xbsIndex_r4/Gateway Out  inherit_from_input=on  hdl_port=off  rows=1  columns=1  UseAsDAC=off  DACChannel='1'  interface=None  automatic_assignment=on  address_offset=hex2dec('00')  intf_name=''  intf_description=''  timing_constraint=None  locs_specified=off  LOCs={}  io_standard={}  block_type=gatewayout
  Inverter : xbsIndex_r4/Inverter  en=off  latency=1  dbl_ovrd=off  block_type=inv
  Logical : xbsIndex_r4/Logical  logical_function=OR  inputs=3  en=off  latency=1  precision=User Defined  arith_type=Boolean  n_bits=16  bin_pt=0  align_bp=on  dbl_ovrd=off  block_type=logical
  Mult : xbsIndex_r4/Mult  precision=User Defined  arith_type="Signed  (2's comp)"  n_bits=32  bin_pt=30  quantization=Truncate  overflow=Saturate  en=off  latency=3  use_behavioral_HDL=off  opt=Speed  use_embedded=on  optimum_pipeline=off  pipeline=on  dbl_ovrd=off  use_rpm=on  placement_style=Triangular  block_type=mult
  Mux : xbsIndex_r4/Mux  inputs=2  en=off  latency=1  precision=Full  arith_type=Unsigned  n_bits=16  bin_pt=14  quantization=Truncate  overflow=Wrap  dbl_ovrd=off  block_type=mux
  Mux1 : xbsIndex_r4/Mux  inputs=2  en=off  latency=1  precision=Full  arith_type=Unsigned  n_bits=16  bin_pt=14  quantization=Truncate  overflow=Wrap  dbl_ovrd=off  block_type=mux
  Mux2 : xbsIndex_r4/Mux  inputs=3  en=off  latency=1  precision=Full  arith_type=Unsigned  n_bits=16  bin_pt=14  quantization=Truncate  overflow=Wrap  dbl_ovrd=off  block_type=mux
  Negate : xbsIndex_r4/Negate  precision=Full  arith_type=Unsigned  n_bits=16  bin_pt=14  quantization=Truncate  overflow=Wrap  en=off  latency=1  dbl_ovrd=off  block_type=negate
  Negate1 : xbsIndex_r4/Negate  precision=Full  arith_type=Unsigned  n_bits=16  bin_pt=14  quantization=Truncate  overflow=Wrap  en=off  latency=1  dbl_ovrd=off  block_type=negate
  Register : xbsIndex_r4/Register  init=0  rst=off  en=on  dbl_ovrd=off  block_type=register
  Register1 : xbsIndex_r4/Register  init=0  rst=off  en=on  dbl_ovrd=off  block_type=register
  Register2 : xbsIndex_r4/Register  init=0  rst=off  en=on  dbl_ovrd=off  block_type=register
  Register3 : xbsIndex_r4/Register  init=0  rst=off  en=off  dbl_ovrd=off  block_type=register
  Relational : xbsIndex_r4/Relational  mode=a=b  op_type=Bool  en=off  latency=0  dbl_ovrd=off  block_type=relational
  Relational1 : xbsIndex_r4/Relational  mode=a=b  op_type=Bool  en=off  latency=0  dbl_ovrd=off  block_type=relational
  Relational2 : xbsIndex_r4/Relational  mode=a=b  op_type=Bool  en=off  latency=0  dbl_ovrd=off  block_type=relational
  Relational3 : xbsIndex_r4/Relational  mode=a>b  op_type=Bool  en=off  latency=1  dbl_ovrd=off  block_type=relational
  Relational4 : xbsIndex_r4/Relational  mode=a<b  op_type=Bool  en=off  latency=1  dbl_ovrd=off  block_type=relational
  Terminator : Terminator
  freqWordDecoder : CryoDetLibCMB/freqWordDecoder
  initial Frequencies1 : Subsystem
  loop filter input : Scope  NumInputPorts=2
  loop filter output : Scope  NumInputPorts=3
  loopFiltervia mcode from old cryodet : Subsystem
  Out1 : Outport
  Out2 : Outport  Port=2
  tag scope: freqBus=global
  wires:
  In2/1 -> Bus Selector/1
  Bus Selector/1 -> initial Frequencies1/1(channel), Relational/1, Gateway Out3/1, Delay3/1  "<channel>"
  Bus Selector/2 -> Mult/1, Register/1  "<freqError>"
  Bus Creator/1 -> Out2/1, [freqBus]
  [fbPolarity] -> Mux/1
  [FBgain] -> Mux/2, Negate/1
  [FBlimit] -> Negate1/1, Mux2/3, Relational4/1
  initial Frequencies1/1(Fi) -> Delay1/1
  Gateway Out13/1 -> Gain1/1
  Gateway Out12/1 -> loop filter output/1
  Gateway Out4/1 -> Gain2/1
  Gateway Out3/1 -> loop filter input/1, Display2/1
  Constant/1 -> Relational/2
  Relational/1 -> Register/2
  Register/1 -> Gateway Out4/1
  Constant1/1 -> Relational1/1
  Relational1/1 -> Register1/2
  Register1/1 -> Gateway Out13/1
  Gain1/1 -> loop filter output/2
  Gain2/1 -> Display3/1, loop filter input/2
  Constant2/1 -> Relational2/1
  Relational2/1 -> Register2/2
  Register2/1 -> Gateway Out5/1
  Gateway Out5/1 -> Gain3/1
  Gain3/1 -> loop filter output/3
  Negate/1 -> Mux/3
  Mult/1 -> AddSub/1
  Mux/1 -> Mult/2
  [fpgaReset] -> Inverter/1
  [FBen] -> Logical/1
  Logical/1 -> Mux1/1
  AddSub/1 -> Mux1/3
  Constant3/1 -> Mux1/2
  Inverter/1 -> Logical/2
  Mux1/1 -> Register3/1, Relational4/2, Relational3/2
  Relational3/1 -> Concat1/1
  Relational4/1 -> Concat1/2
  Concat1/1 -> Mux2/1
  Negate1/1 -> Mux2/4, Relational3/1
  Register3/1 -> Mux2/2
  Delay/1 -> AddSub/2
  Mux2/1 -> AddSub1/1, Delay/1
  freqWordDecoder/2 -> Terminator/1
  freqWordDecoder/1 -> Logical/3
  Delay3/1 -> Delay2/1
  Delay2/1 -> Delay4/1
  Delay4/1 -> Delay5/1
  Delay5/1 -> Delay6/1
  freqWordDecoder/3 -> Delay7/1
  Delay1/1 -> freqWordDecoder/1
  Delay7/1 -> Delay9/1
  Delay9/1 -> Delay10/1
  Delay10/1 -> Relational2/2, Gateway Out12/1, Relational1/2, AddSub1/2  "Finitial"
  AddSub1/1 -> Register2/1, Register1/1, Bus Creator/2  "Fi"
  Delay6/1 -> Bus Creator/1  "channel"
